simulink model "MLI"  (R2023a)
settings: Solver=VariableStepAuto  StartTime=0.0  StopTime=5  RelTol=1e-3
libraries: spsMosfetLib x8, simulink x4, spsDCVoltageSourceLib x2, spsVoltageMeasurementLib x2, spsSeriesRLCLoadLib x1, sps_lib x1
settings Model: Creator=USER  LastModifiedBy=USER

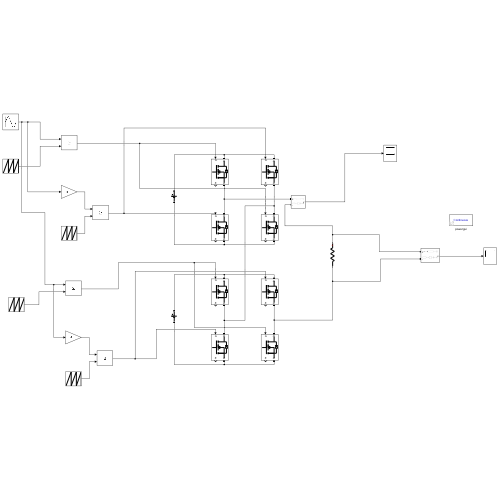
[thumbnail: Simulink's stored preview of the top-level diagram]
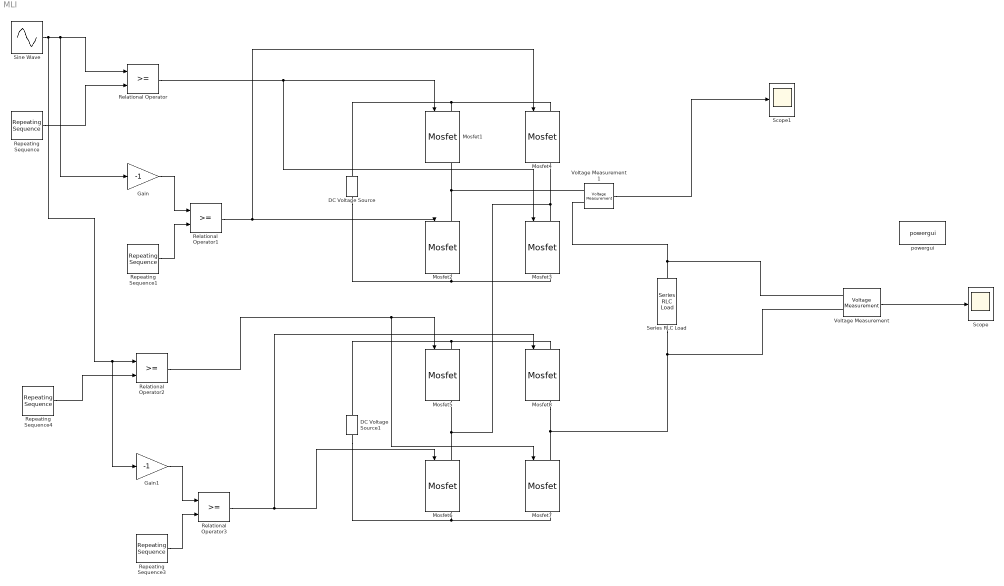
== system MLI ==
  DC Voltage Source : spsDCVoltageSourceLib/DC Voltage Source  Amplitude=100  Measurements=None
  DC Voltage Source1 : spsDCVoltageSourceLib/DC Voltage Source  Amplitude=100  Measurements=None
  Gain : Gain  Gain=-1
  Gain1 : Gain  Gain=-1
  Mosfet{1..8} (8 alike) : spsMosfetLib/Mosfet  Ron=0.1  Lon=0  Rd=0.01  Vfd=0  IC=0  Rs=1e5  Cs=inf  Measurements=on
  Relational Operator{,1..3} (4 alike) : RelationalOperator  OutDataTypeStr=boolean  RndMeth=Simplest  InputSameDT=off
  Repeating Sequence : simulink/Sources/Repeating Sequence  rep_seq_t=[0 1]  rep_seq_y=[0 1]
  Repeating Sequence1 : simulink/Sources/Repeating Sequence  rep_seq_t=[0 1]  rep_seq_y=[0 1]
  Repeating Sequence3 : simulink/Sources/Repeating Sequence  rep_seq_t=[0 1]  rep_seq_y=[1 2]
  Repeating Sequence4 : simulink/Sources/Repeating Sequence  rep_seq_t=[0 1]  rep_seq_y=[0 1]
  Scope : Scope
  Scope1 : Scope
  Series RLC Load : spsSeriesRLCLoadLib/Series RLC Load  LConnTagsString=a  RConnTagsString=__new0  NominalVoltage=1000  NominalFrequency=60  ActivePower=10e3  InductivePower=0  CapacitivePower=0  Setx0=off  InitialVoltage=0  SetiL0=off  InitialCurrent=0  Measurements=None  LoadType=constant Z
  Sine Wave : Sin  Amplitude=2  Frequency=2*pi*50  SampleTime=0
  Voltage Measurement : spsVoltageMeasurementLib/Voltage Measurement  PhasorSimulation=off  OutputType=Complex  PSBequivalent=0
  Voltage Measurement1 : spsVoltageMeasurementLib/Voltage Measurement  PhasorSimulation=off  OutputType=Complex  PSBequivalent=0
  powergui : sps_lib/powergui  Priority=1  SimulationMode=Continuous  SampleTime=50e-6  frequency=60  Iterations=50  frequencyindice=0  Pbase=100e6  ErrMax=1e-4  UnitsV=kV  UnitsW=MW  buscounter=0  FunctionMessages=off  echomessages=off  EnableUseOfTLC=off  CurrentSourceSwitches=off  DisableSnubberDevices=off  DisableRonSwitches=off  DisableVfSwitches=off  DisplayEquations=off  AutomaticDiscreteSolvers=off  SolverType=Tustin/Backward Euler (TBE)  Interpol=off  ExternalGateDelay=off  methode=off  Ts=100  x0status=blocks  SPID=on  SwTol=0  HookPort=off  NonlinearTolerance=1e-4  nMaxIteration=100  ContinueOnMaxIteration=off  RestoreLinks=warning  ResistiveCurrentMeasurement=off  Frange=[0:2:500]  Ylog=off  Xlog=on  ShowGrid=off  save=off  variable=ZData  structure=0  ZoomFFT=off  StartTime=0.0  cycles=1  DisplayStyle=1  fundamental=60  FreqAxis=off  MaxFrequency=1000  frequencyindicesteady=1  RmsSteady=1  display=off
  wires:
  Sine Wave/1 -> Gain1/1, Relational Operator2/1, Gain/1, Relational Operator/1
  Voltage Measurement/1 -> Scope/1
  Repeating Sequence3/1 -> Relational Operator3/2
  Gain1/1 -> Relational Operator3/1
  Repeating Sequence/1 -> Relational Operator/2
  Gain/1 -> Relational Operator1/1
  Relational Operator2/1 -> Mosfet7/1, Mosfet5/1
  Repeating Sequence1/1 -> Relational Operator1/2
  Relational Operator3/1 -> Mosfet6/1, Mosfet8/1
  Relational Operator/1 -> Mosfet3/1, Mosfet1/1
  Relational Operator1/1 -> Mosfet4/1, Mosfet2/1
  Voltage Measurement1/1 -> Scope1/1
  Repeating Sequence4/1 -> Relational Operator2/2
  connections:
  Series RLC Load/RConn1 -- Voltage Measurement/LConn2 -- Mosfet7/LConn1 -- Mosfet8/RConn1
  Mosfet6/RConn1 -- Mosfet7/RConn1 -- DC Voltage Source1/LConn1
  Mosfet2/RConn1 -- Mosfet3/RConn1 -- DC Voltage Source/LConn1
  Series RLC Load/LConn1 -- Voltage Measurement1/LConn2 -- Voltage Measurement/LConn1
  Mosfet1/LConn1 -- Mosfet4/LConn1 -- DC Voltage Source/RConn1
  Mosfet6/LConn1 -- Mosfet4/RConn1 -- Mosfet3/LConn1 -- Mosfet5/RConn1
  Mosfet5/LConn1 -- Mosfet8/LConn1 -- DC Voltage Source1/RConn1
  Mosfet2/LConn1 -- Voltage Measurement1/LConn1 -- Mosfet1/RConn1
